simulink model "ChiefMaster_TTC580"  (R2022b)
settings: Solver=FixedStepAuto  StartTime=0.0  StopTime=10  FixedStep=0.01  RelTol=1e-3
values from neighbouring files (symbols this model uses):
  BattBox1_No = single(1)    [Parameters.m]
  BattBox2_No = single(2)    [Parameters.m]
  BattBox3_No = single(3)    [Parameters.m]
  CurrentLB = single(-3)    [Parameters.m]
  CurrentReductionConstant_Lvl0 = single(0.03)    [Parameters.m]
  CurrentReductionConstant_Lvl1 = single(0.05)    [Parameters.m]
  CurrentReductionConstant_Lvl2 = single(0.07)    [Parameters.m]
  CurrentReductionConstant_Lvl3 = single(0.1)    [Parameters.m]
  CurrentUB = single(3)    [Parameters.m]
  DCHV_Minus_In_Delay_ms = single(500)    [Parameters.m]
  FL_sHVC_CellBalanceVoltage_mV = single(3500)    [Parameters.m]
  FL_sInrushCurrent_dividebyzero = single(0.00001)    [Parameters.m]
  FL_u8HMI_BuzzerTimer = uint8(3)    [Parameters.m]
  IP_boActValue = true    [Parameters.m]
  IP_boDeactValue = false    [Parameters.m]
  IP_boInitValue = false    [Parameters.m]
  IP_s_LB = 18000    [Parameters.m]
  IP_s_UB = 22000    [Parameters.m]
  IP_sBatt1_ChargeCurrentMax_Factor = single(0.1)    [Parameters.m]
  IP_sBatt1_ChargeCurrentMax_LB = single(0)    [Parameters.m]
  IP_sBatt1_ChargeCurrentMax_Offset = single(0)    [Parameters.m]
  IP_sBatt1_ChargeCurrentMax_UB = single(6553.5)    [Parameters.m]
  IP_sBatt1_Current_Factor = single(0.1)    [Parameters.m]
  IP_sBatt1_Current_LB = single(-3276.8)    [Parameters.m]
  IP_sBatt1_Current_Offset = single(0)    [Parameters.m]
  IP_sBatt1_Current_UB = single(3276.8)    [Parameters.m]
  IP_sBatt1_DisChargeCurrentMax_Factor = single(0.1)    [Parameters.m]
  IP_sBatt1_DisChargeCurrentMax_LB = single(0)    [Parameters.m]
  IP_sBatt1_DisChargeCurrentMax_Offset = single(0)    [Parameters.m]
  IP_sBatt1_DisChargeCurrentMax_UB = single(6553.5)    [Parameters.m]
  IP_sBatt1_InsulationResistance_Factor = single(5)    [Parameters.m]
  IP_sBatt1_InsulationResistance_LB = single(0)    [Parameters.m]
  IP_sBatt1_InsulationResistance_Offset = single(0)    [Parameters.m]
  IP_sBatt1_InsulationResistance_UB = single(0)    [Parameters.m]
  IP_sBatt1_LiBa_IntResist_mOhm = single(25)    [Parameters.m]
  IP_sBatt1_SOC_Factor = single(1)    [Parameters.m]
  IP_sBatt1_SOC_LB = single(0)    [Parameters.m]
  IP_sBatt1_SOC_Offset = single(0)    [Parameters.m]
  IP_sBatt1_SOC_UB = single(100)    [Parameters.m]
  IP_sBatt1_SOH_Factor = single(1)    [Parameters.m]
  IP_sBatt1_SOH_LB = single(0)    [Parameters.m]
  IP_sBatt1_SOH_Offset = single(0)    [Parameters.m]
  IP_sBatt1_SOH_UB = single(100)    [Parameters.m]
  IP_sBatt1_Ubatt_Factor = single(0.1)    [Parameters.m]
  IP_sBatt1_Ubatt_LB = single(0)    [Parameters.m]
  IP_sBatt1_Ubatt_Offset = single(0)    [Parameters.m]
  IP_sBatt1_Ubatt_UB = single(6553.5)    [Parameters.m]
  IP_sBatt1_UserRi_Factor = single(1)    [Parameters.m]
  IP_sBatt1_UserRi_LB = single(0)    [Parameters.m]
  IP_sBatt1_UserRi_Offset = single(0)    [Parameters.m]
  IP_sBatt1_UserRi_UB = single(255)    [Parameters.m]
  IP_sBatt1_VoltageAtSensor_Factor = single(0.02)    [Parameters.m]
  IP_sBatt1_VoltageAtSensor_LB = single(0)    [Parameters.m]
  IP_sBatt1_VoltageAtSensor_Offset = single(0)    [Parameters.m]
  IP_sBatt1_VoltageAtSensor_UB = single(1310.7)    [Parameters.m]
  IP_sBatt2_LiBa_IntResist_mOhm = single(25)    [Parameters.m]
  IP_sBatt3_LiBa_IntResist_mOhm = single(25)    [Parameters.m]
  IP_sEM_LB = 2000    [Parameters.m]
  IP_sEM_UB = 8000    [Parameters.m]
  IP_sFB_LB = 5000    [Parameters.m]
  IP_sFB_UB = 10000    [Parameters.m]
  IP_sHVIL_LB = 12000    [Parameters.m]
  IP_sHVIL_UB = 15000    [Parameters.m]
  IP_sLoad_Voltage_Factor = single(1)    [Parameters.m]
  IP_sLoad_Voltage_LB = single(0)    [Parameters.m]
  IP_sLoad_Voltage_Offset = single(0)    [Parameters.m]
  IP_sLoad_Voltage_UB = single(65535)    [Parameters.m]
  IP_u8HVIL_Delay_ms = uint8(100)    [Parameters.m]
  IP_u8HW_IN_delay_ms = uint8(100)    [Parameters.m]
  IT_sInsulationSafeValue_kOhm = single(650)    [Parameters.m]
  IT_u8IMD_DelayTime_s = uint8(20)    [Parameters.m]
  MainHV_Minus_In_Delay = single(5)    [Parameters.m]
  MainHV_StatusDelay = single(5)    [Parameters.m]
  NotAvailable_uint16 = single(65535)    [Parameters.m]
  NotAvailable_uint8 = uint8(255)    [Parameters.m]
  OP_boHVIL_Supply = boolean(1)    [Parameters.m]
  SafeCurrentToCloseHV_A = single(5)    [Parameters.m]
  SafeVoltageToCloseHV_V = single(0.5)    [Parameters.m]
  UnexpectedBattChargingFcn_Available = boolean(1)    [Parameters.m]
  Voltage_NA_UB = uint16(65535)    [Parameters.m]
  VoltageSensorAvailableBB1 = boolean(0)    [Parameters.m]
  VoltageSensorAvailableBB2 = boolean(0)    [Parameters.m]
  VoltageSensorAvailableBB3 = boolean(0)    [Parameters.m]
libraries: simulink x184, Library_DataProcessing_v1_1 x167, Library_DataProcessing_v1 x142, libCM x28
(part 10 of 19)

== system ChiefMaster_TTC580/ChiefMaster/Flow Logic/System Status/SDError/Subsystem ==
  KL15_Reset : Inport
  BattPack_REL_Databus : Inport  Port=2
  BatteryPackSignals : Inport  Port=3
  AND : Logic  Inputs=3  AllPortsSameDT=off  OutDataTypeStr=boolean
  AND1 : Logic  Inputs=3  AllPortsSameDT=off  OutDataTypeStr=boolean
  AND2 : Logic  Inputs=3  AllPortsSameDT=off  OutDataTypeStr=boolean
  Bus Selector : BusSelector  OutputSignals=IT_BatterySignal_Databus.IT_sBMS_Current_BB1,IT_BatterySignal_Databus.IT_sBMS_Current_BB2,IT_BatterySignal_Databus.IT_sBMS_Current_BB3,IT_BatterySignal_Databus.IT_boBMS_SDError_BB1,IT_BatterySignal_Databus.IT_boBMS_SDError_BB2,IT_BatterySignal_Databus.IT_boBMS_SDError_BB3
  Bus Selector1 : BusSelector  OutputSignals=FL_boREQ_HV_ON_BB1,FL_boREQ_HV_ON_BB2,FL_boREQ_HV_ON_BB3
  Chart : Stateflow chart  TreatAsAtomicUnit=on
  Chart1 : Stateflow chart  TreatAsAtomicUnit=on
  Chart2 : Stateflow chart  TreatAsAtomicUnit=on
  Compare To Constant1 : simulink/Logic and Bit Operations/Compare To Constant  relop=>  const=1  OutDataTypeStr=boolean
  Compare To Constant2 : simulink/Logic and Bit Operations/Compare To Constant  relop===  const=0  OutDataTypeStr=boolean
  Compare To Constant3 : simulink/Logic and Bit Operations/Compare To Constant  relop=>  const=1  OutDataTypeStr=boolean
  Compare To Constant4 : simulink/Logic and Bit Operations/Compare To Constant  relop===  const=0  OutDataTypeStr=boolean
  Compare To Constant5 : simulink/Logic and Bit Operations/Compare To Constant  relop=>  const=1  OutDataTypeStr=boolean
  Compare To Constant6 : simulink/Logic and Bit Operations/Compare To Constant  relop===  const=0  OutDataTypeStr=boolean
  Detect Decrease : simulink/Logic and Bit Operations/Detect Decrease  vinit=0.0  OutDataTypeStr=boolean
  Detect Decrease1 : simulink/Logic and Bit Operations/Detect Decrease  vinit=0.0  OutDataTypeStr=boolean
  Detect Decrease2 : simulink/Logic and Bit Operations/Detect Decrease  vinit=0.0  OutDataTypeStr=boolean
  OR : Logic  Operator=OR  Inputs=3  AllPortsSameDT=off  OutDataTypeStr=boolean
  REL_Error_BB : Outport
  wires:
  BattPack_REL_Databus/1 -> Bus Selector1/1
  Bus Selector/1 -> Compare To Constant1/1  "<IT_sBMS_Current_BB1>"
  BatteryPackSignals/1 -> Bus Selector/1
  Compare To Constant6/1 -> Chart2/2(REQ_HV_ON_BB)
  Compare To Constant4/1 -> Chart1/2(REQ_HV_ON_BB)
  Compare To Constant2/1 -> Chart/2(REQ_HV_ON_BB)
  OR/1 -> REL_Error_BB/1
  AND2/1 -> OR/3
  AND1/1 -> OR/2
  KL15_Reset/1 -> Chart/3(KL15_CM_Reset), Chart1/3(KL15_CM_Reset), Chart2/3(KL15_CM_Reset)
  Chart2/1(Out) -> AND2/3
  Detect Decrease2/1 -> Chart2/1(In)
  Compare To Constant5/1 -> AND2/1
  Bus Selector/3 -> Compare To Constant5/1  "<IT_sBMS_Current_BB3>"
  Bus Selector/6 -> AND2/2  "<IT_boBMS_SDError_BB3>"
  Bus Selector1/3 -> Detect Decrease2/1, Compare To Constant6/1  "<FL_boREQ_HV_ON_BB3>"
  Bus Selector1/2 -> Compare To Constant4/1, Detect Decrease1/1  "<FL_boREQ_HV_ON_BB2>"
  Bus Selector/5 -> AND1/2  "<IT_boBMS_SDError_BB2>"
  Bus Selector/2 -> Compare To Constant3/1  "<IT_sBMS_Current_BB2>"
  Compare To Constant3/1 -> AND1/1
  Detect Decrease1/1 -> Chart1/1(In)
  Chart1/1(Out) -> AND1/3
  AND/1 -> OR/1
  Chart/1(Out) -> AND/3
  Detect Decrease/1 -> Chart/1(In)
  Compare To Constant1/1 -> AND/1
  Bus Selector/4 -> AND/2  "<IT_boBMS_SDError_BB1>"
  Bus Selector1/1 -> Compare To Constant2/1, Detect Decrease/1  "<FL_boREQ_HV_ON_BB1>"

== system ChiefMaster_TTC580/ChiefMaster/Flow Logic/System Status/SDError/Subsystem6 ==
  BatteryPackSignals : Inport
  AND3 : Logic  Operator=OR  Inputs=3  AllPortsSameDT=off  OutDataTypeStr=boolean
  Bus Selector2 : BusSelector  OutputSignals=IT_HW_Input_Databus.IT_boHW_Proximity_BB1,IT_HW_Input_Databus.IT_boHW_Proximity_BB2,IT_HW_Input_Databus.IT_boHW_Proximity_BB3
  Compare To Constant : simulink/Logic and Bit Operations/Compare To Constant  relop===  const=0  OutDataTypeStr=boolean
  Compare To Constant1 : simulink/Logic and Bit Operations/Compare To Constant  relop===  const=0  OutDataTypeStr=boolean
  Compare To Constant2 : simulink/Logic and Bit Operations/Compare To Constant  relop===  const=0  OutDataTypeStr=boolean
  SecuritySwitchError : Outport
  wires:
  Bus Selector2/2 -> Compare To Constant1/1  "<IT_boHW_Proximity_BB2>"
  AND3/1 -> SecuritySwitchError/1
  Bus Selector2/3 -> Compare To Constant2/1  "<IT_boHW_Proximity_BB3>"
  BatteryPackSignals/1 -> Bus Selector2/1
  Bus Selector2/1 -> Compare To Constant/1  "<IT_boHW_Proximity_BB1>"
  Compare To Constant/1 -> AND3/1
  Compare To Constant1/1 -> AND3/2
  Compare To Constant2/1 -> AND3/3

== system ChiefMaster_TTC580/ChiefMaster/Input Processing/Actia/Batt Box 1/Subsystem1 ==
  C_Batt1_ADS_3_560 : Inport
  C_Batt1_ADS_3_560_Timeout : Inport  Port=2
  Demux : Demux  Outputs=8
  Subsystem3 : Subsystem
  Terminator{,1..5} (6 alike) : Terminator
  IP_sActia_Batt1_Ubatt_Databus : Outport
  wires:
  C_Batt1_ADS_3_560/1 -> Demux/1
  Demux/2 -> Subsystem3/1(byte1)
  Demux/3 -> Subsystem3/2(byte2)
  Subsystem3/1(IP_sBatt1_Ubatt_Databus) -> IP_sActia_Batt1_Ubatt_Databus/1  "IP_sActia_Batt1_Ubatt_Databus"
  Demux/8 -> Terminator/1
  C_Batt1_ADS_3_560_Timeout/1 -> Subsystem3/3(C_Batt1_ADS_3_560_Timeout)
  Demux/7 -> Terminator1/1
  Demux/6 -> Terminator2/1
  Demux/5 -> Terminator3/1
  Demux/4 -> Terminator4/1
  Demux/1 -> Terminator5/1

== system ChiefMaster_TTC580/ChiefMaster/Input Processing/Actia/Batt Box 1/Subsystem13 ==
  C_Batt1_MyStatus_140_Timeout : Inport
  C_Batt1_Error_100_Timeout : Inport  Port=2
  C_Batt1_ADS_8_600_Timeout : Inport  Port=3
  C_Batt1_ADS_0_500_Timeout : Inport  Port=4
  C_Batt1_ADS_1_520_Timeout : Inport  Port=5
  C_Batt1_ADS_3_560_Timeout : Inport  Port=6
  AND : Logic  Inputs=6  AllPortsSameDT=off  OutDataTypeStr=boolean
  Constant : Constant
  Constant1 : Constant  Value=0
  NOT{,1..5} (6 alike) : Logic  Operator=NOT  AllPortsSameDT=off  OutDataTypeStr=boolean
  Switch : Switch  Criteria=u2 > Threshold  SaturateOnIntegerOverflow=off  InputSameDT=off
  IP_sActia_Batt1_Availability : Outport
  wires:
  Constant1/1 -> Switch/3
  Constant/1 -> Switch/1
  AND/1 -> Switch/2
  NOT4/1 -> AND/6
  NOT3/1 -> AND/5
  NOT2/1 -> AND/3
  NOT1/1 -> AND/2
  NOT/1 -> AND/1
  C_Batt1_ADS_1_520_Timeout/1 -> NOT3/1
  C_Batt1_ADS_8_600_Timeout/1 -> NOT2/1
  C_Batt1_Error_100_Timeout/1 -> NOT1/1
  C_Batt1_MyStatus_140_Timeout/1 -> NOT/1
  Switch/1 -> IP_sActia_Batt1_Availability/1  "IP_sActia_Batt1_Availability"
  C_Batt1_ADS_3_560_Timeout/1 -> NOT4/1
  C_Batt1_ADS_0_500_Timeout/1 -> NOT5/1
  NOT5/1 -> AND/4

== system ChiefMaster_TTC580/ChiefMaster/Input Processing/Actia/Batt Box 1/Subsystem2 ==
  C_Actia_Batt1_MyStatus_Msg : Inport
  C_Actia_Batt1_MyStatus_Timeout : Inport  Port=2
  Demux : Demux  Outputs=8
  NOT : Logic  Priority=5520  Operator=NOT  AllPortsSameDT=off  OutDataTypeStr=boolean
  Subsystem : Subsystem
  Subsystem2 : Subsystem
  Subsystem3 : Subsystem
  Subsystem4 : Subsystem
  Terminator : Terminator
  Batt1_MyStatus1_Databus : Outport
  IP_sActia_Batt1_ChargeCurrentMax_A_Databus : Outport  Port=2
  IP_sActia_Batt1_DisChargeCurrentMax_A_Databus : Outport  Port=3
  IP_sActia_Batt1_VoltageAtSensor_V_Databus : Outport  Port=4
  wires:
  C_Actia_Batt1_MyStatus_Msg/1 -> Demux/1
  Demux/1 -> Subsystem/1(byte1)
  Subsystem/1(Batt1_MyStatus1_Databus) -> Batt1_MyStatus1_Databus/1  "IP_Actia_Batt1_MyStatus1_Databus"
  Demux/2 -> Subsystem4/1(byte2)
  Demux/3 -> Subsystem4/2(byte3)
  Demux/4 -> Subsystem2/1(byte2)
  Demux/5 -> Subsystem2/2(byte3)
  Demux/6 -> Subsystem3/1(byte2)
  Demux/7 -> Subsystem3/2(byte3)
  Subsystem4/1(IP_sBatt1_ChargeCurrentMax_A_Databus) -> IP_sActia_Batt1_ChargeCurrentMax_A_Databus/1  "IP_sActia_Batt1_ChargeCurrentMax_A_Databus"
  Subsystem2/1(IP_sBatt1_DisChargeCurrentMax_A_Databus) -> IP_sActia_Batt1_DisChargeCurrentMax_A_Databus/1  "IP_sActia_Batt1_DisChargeCurrentMax_A_Databus"
  Subsystem3/1(IP_sBatt1_VoltageAtSensor_V_Databus) -> IP_sActia_Batt1_VoltageAtSensor_V_Databus/1  "IP_sActia_Batt1_VoltageAtSensor_V_Databus"
  Demux/8 -> Terminator/1
  C_Actia_Batt1_MyStatus_Timeout/1 -> NOT/1, Subsystem3/3(C_Actia_Batt1_MyStatus_Timeout), Subsystem2/3(C_Actia_Batt1_MyStatus_Timeout), Subsystem4/3(C_Actia_Batt1_MyStatus_Timeout)
  NOT/1 -> Subsystem/Enable

== system ChiefMaster_TTC580/ChiefMaster/Input Processing/Actia/Batt Box 1/Subsystem3 ==
  C_Batt1_ADS_0_500 : Inport
  C_Batt1_ADS_0_500_Timeout : Inport  Port=2
  Demux : Demux  Outputs=8
  Subsystem1 : Subsystem
  Subsystem2 : Subsystem
  Terminator{1..4} (4 alike) : Terminator
  IP_sActia_Batt1_MinCellVolt_mV_DataBus : Outport
  IP_sActia_Batt1_MaxCellVolt_mV_DataBus : Outport  Port=2
  wires:
  Subsystem2/1(IP_sActia_Batt1_MaxCellVolt_mV_DataBus) -> IP_sActia_Batt1_MaxCellVolt_mV_DataBus/1
  Subsystem1/1(IP_sActia_Batt1_MinCellVolt_mV_DataBus) -> IP_sActia_Batt1_MinCellVolt_mV_DataBus/1
  Demux/7 -> Subsystem2/2(byte7)
  Demux/6 -> Subsystem2/1(byte6)
  Demux/5 -> Subsystem1/2(byte5)
  Demux/4 -> Subsystem1/1(byte4)
  C_Batt1_ADS_0_500/1 -> Demux/1
  Demux/1 -> Terminator1/1
  Demux/2 -> Terminator2/1
  Demux/3 -> Terminator3/1
  C_Batt1_ADS_0_500_Timeout/1 -> Subsystem1/3(C_BMS500_Timeout), Subsystem2/3(C_BMS500_Timeout)
  Demux/8 -> Terminator4/1

== system ChiefMaster_TTC580/ChiefMaster/Input Processing/Actia/Batt Box 1/Subsystem4 ==
  C_Actia_Batt1_Error : Inport
  C_Actia_Batt1_Error_Timeout : Inport  Port=2
  Bus Creator : BusCreator  Inputs=7
  Bus Creator1 : BusCreator  Inputs=1
  Demux : Demux  Outputs=8
  NOT : Logic  Priority=5520  Operator=NOT  AllPortsSameDT=off  OutDataTypeStr=boolean
  Subsystem : Subsystem
  Subsystem1 : Subsystem
  Subsystem2 : Subsystem
  Terminator{1,3..6} (5 alike) : Terminator
  IP_Actia_sBatt1_MyStatus2_Databus : Outport
  IP_Actia_Batt1_Error_Databus : Outport  Port=2
  wires:
  Demux/8 -> Subsystem1/1(byte8)
  Bus Creator/1 -> IP_Actia_sBatt1_MyStatus2_Databus/1  "Batt1_MyStatus2_Databus"
  Demux/7 -> Subsystem/1(byte7)
  C_Actia_Batt1_Error/1 -> Demux/1
  Demux/1 -> Terminator1/1
  Demux/2 -> Subsystem2/1(byte2)
  Demux/3 -> Terminator3/1
  Demux/4 -> Terminator4/1
  Demux/5 -> Terminator5/1
  Demux/6 -> Terminator6/1
  C_Actia_Batt1_Error_Timeout/1 -> NOT/1
  NOT/1 -> Subsystem/Enable, Subsystem1/Enable, Subsystem2/Enable
  Subsystem/1(IP_boBatt1_HV_relay_PLUS_Sense) -> Bus Creator/1
  Subsystem/2(IP_boBatt1_HV_PRECHARGE_active) -> Bus Creator/2
  Subsystem/3(IP_boBatt1_HV_relay_MINUS_Sense) -> Bus Creator/3
  Subsystem/4(IP_boBatt1_IMD_active) -> Bus Creator/4
  Subsystem1/1(IP_boBatt1_Drive_Mode_active) -> Bus Creator/5
  Subsystem1/2(IP_boBatt1_PlugIn_Mode_active) -> Bus Creator/6
  Subsystem1/3(IP_boBatt1_Charging_finished) -> Bus Creator/7
  Subsystem2/1(IP_boBatt1_SDErr_SecuritySwitch) -> Bus Creator1/1
  Bus Creator1/1 -> IP_Actia_Batt1_Error_Databus/1  "Batt1_Error_Databus"

== system ChiefMaster_TTC580/ChiefMaster/Input Processing/Actia/Batt Box 1/Subsystem5 ==
  C_Batt1_ADS_8_600 : Inport
  C_Batt1_ADS_8_600_Timeout : Inport  Port=2
  Demux : Demux  Outputs=8
  Subsystem : Subsystem
  Subsystem1 : Subsystem
  Subsystem2 : Subsystem
  Subsystem3 : Subsystem
  Terminator1 : Terminator
  Terminator2 : Terminator
  Terminator3 : Terminator
  IP_sActia_Batt1_Current_A_DataBus : Outport
  IP_sActia_Batt1_InsulationResistance_kOhms_DataBus : Outport  Port=2
  IP_sActia_Batt1_SOC_percent_DataBus : Outport  Port=3
  IP_sActia_Batt1_SOH_percent_DataBus : Outport  Port=4
  wires:
  Demux/8 -> Subsystem3/1(byte8)
  Subsystem/1(IP_sBatt1_InsulationResistance_kOhms_DataBus) -> IP_sActia_Batt1_InsulationResistance_kOhms_DataBus/1  "IP_sActia_Batt1_InsulationResistance_kOhms_DataBus"
  Subsystem2/1(IP_sBatt1_Current_A_DataBus) -> IP_sActia_Batt1_Current_A_DataBus/1  "IP_sActia_Batt1_Current_A_DataBus"
  Demux/6 -> Subsystem/1(byte6)
  Demux/5 -> Subsystem2/2(byte5)
  Demux/4 -> Subsystem2/1(byte4)
  C_Batt1_ADS_8_600/1 -> Demux/1
  Demux/1 -> Terminator1/1
  Demux/2 -> Terminator2/1
  Demux/3 -> Terminator3/1
  C_Batt1_ADS_8_600_Timeout/1 -> Subsystem3/2(C_Batt1_ADS_8_600_Timeout), Subsystem1/2(C_Batt1_ADS_8_600_Timeout), Subsystem/2(C_Batt1_ADS_8_600_Timeout), Subsystem2/3(C_Batt1_ADS_8_600_Timeout)
  Demux/7 -> Subsystem1/1(byte7)
  Subsystem1/1(IP_sBatt1_SOC_percent_DataBus) -> IP_sActia_Batt1_SOC_percent_DataBus/1  "IP_sActia_Batt1_SOC_percent_DataBus"
  Subsystem3/1(IP_sBatt1_SOH_percent_DataBus) -> IP_sActia_Batt1_SOH_percent_DataBus/1  "IP_sActia_Batt1_SOH_percent_DataBus"

== system ChiefMaster_TTC580/ChiefMaster/Input Processing/Actia/Batt Box 1/Subsystem6 ==
  C_Batt1_ADS_1_520 : Inport
  C_Batt1_ADS_1_520_Timeout : Inport  Port=2
  Demux : Demux  Outputs=8
  Subsystem1 : Subsystem
  Subsystem2 : Subsystem
  Subsystem3 : Subsystem
  Terminator1 : Terminator
  Terminator2 : Terminator
  Terminator3 : Terminator
  IP_sActia_Batt1_UserRi_mOhms_DataBus : Outport
  IP_sActia_Batt1_MinTemp_degC_DataBus : Outport  Port=2
  IP_sActia_Batt1_MaxTemp_degC_DataBus : Outport  Port=3
  wires:
  Subsystem3/1(IP_sBatt1_UserRi_mOhms_DataBus) -> IP_sActia_Batt1_UserRi_mOhms_DataBus/1  "IP_sActia_Batt1_UserRi_mOhms_DataBus"
  C_Batt1_ADS_1_520_Timeout/1 -> Subsystem3/2(C_Batt1_ADS_8_600_Timeout), Subsystem2/3(C_BMS214_Timeout), Subsystem1/3(C_BMS214_Timeout)
  Demux/3 -> Terminator3/1
  Demux/2 -> Terminator2/1
  Demux/1 -> Terminator1/1
  C_Batt1_ADS_1_520/1 -> Demux/1
  Demux/8 -> Subsystem3/1(byte8)
  Demux/4 -> Subsystem1/1(byte4)
  Demux/5 -> Subsystem1/2(byte5)
  Demux/6 -> Subsystem2/1(byte6)
  Demux/7 -> Subsystem2/2(byte7)
  Subsystem1/1(IP_sBMS_MinTemp_degC_DataBus) -> IP_sActia_Batt1_MinTemp_degC_DataBus/1
  Subsystem2/1(IP_sBMS_MaxTemp_degC_DataBus) -> IP_sActia_Batt1_MaxTemp_degC_DataBus/1

== system ChiefMaster_TTC580/ChiefMaster/Input Processing/Actia/Batt Box 2/Subsystem1 ==
  C_Batt2_ADS_3_560 : Inport
  C_Batt2_ADS_3_560_Timeout : Inport  Port=2
  Demux : Demux  Outputs=8
  Subsystem3 : Subsystem
  Terminator{,1..5} (6 alike) : Terminator
  IP_sActia_Batt2_Ubatt_Databus : Outport
  wires:
  Demux/1 -> Terminator5/1
  Demux/4 -> Terminator4/1
  Demux/5 -> Terminator3/1
  Demux/6 -> Terminator2/1
  Demux/7 -> Terminator1/1
  C_Batt2_ADS_3_560_Timeout/1 -> Subsystem3/3(C_Batt2_ADS_3_560_Timeout)
  Demux/8 -> Terminator/1
  Subsystem3/1(IP_sBatt2_Ubatt_Databus) -> IP_sActia_Batt2_Ubatt_Databus/1  "IP_sActia_Batt2_Ubatt_Databus"
  Demux/3 -> Subsystem3/2(byte2)
  Demux/2 -> Subsystem3/1(byte1)
  C_Batt2_ADS_3_560/1 -> Demux/1

== system ChiefMaster_TTC580/ChiefMaster/Input Processing/Actia/Batt Box 2/Subsystem13 ==
  C_Batt2_MyStatus_140_Timeout : Inport
  C_Batt2_Error_100_Timeout : Inport  Port=2
  C_Batt2_ADS_8_600_Timeout : Inport  Port=3
  C_Batt2_ADS_501_Timeout : Inport  Port=4
  C_Batt2_ADS_1_520_Timeout : Inport  Port=5
  C_Batt2_ADS_3_560_Timeout : Inport  Port=6
  AND : Logic  Inputs=6  AllPortsSameDT=off  OutDataTypeStr=boolean
  Constant : Constant
  Constant1 : Constant  Value=0
  NOT{,1..5} (6 alike) : Logic  Operator=NOT  AllPortsSameDT=off  OutDataTypeStr=boolean
  Switch : Switch  Criteria=u2 > Threshold  SaturateOnIntegerOverflow=off  InputSameDT=off
  IP_sActia_Batt2_Availability : Outport
  wires:
  C_Batt2_ADS_3_560_Timeout/1 -> NOT4/1
  Switch/1 -> IP_sActia_Batt2_Availability/1  "IP_sActia_Batt2_Availability"
  C_Batt2_MyStatus_140_Timeout/1 -> NOT/1
  C_Batt2_Error_100_Timeout/1 -> NOT1/1
  C_Batt2_ADS_8_600_Timeout/1 -> NOT2/1
  C_Batt2_ADS_1_520_Timeout/1 -> NOT3/1
  NOT/1 -> AND/1
  NOT1/1 -> AND/2
  NOT2/1 -> AND/3
  NOT3/1 -> AND/5
  NOT4/1 -> AND/6
  AND/1 -> Switch/2
  Constant/1 -> Switch/1
  Constant1/1 -> Switch/3
  C_Batt2_ADS_501_Timeout/1 -> NOT5/1
  NOT5/1 -> AND/4

== system ChiefMaster_TTC580/ChiefMaster/Input Processing/Actia/Batt Box 2/Subsystem2 ==
  C_Actia_Batt2_MyStatus_Msg : Inport
  C_Actia_Batt2_MyStatus_Timeout : Inport  Port=2
  Demux : Demux  Outputs=8
  NOT : Logic  Priority=5520  Operator=NOT  AllPortsSameDT=off  OutDataTypeStr=boolean
  Subsystem : Subsystem
  Subsystem2 : Subsystem
  Subsystem3 : Subsystem
  Subsystem4 : Subsystem
  Terminator : Terminator
  Batt2_MyStatus1_Databus : Outport
  IP_sActia_Batt2_ChargeCurrentMax_A_Databus : Outport  Port=2
  IP_sActia_Batt2_DisChargeCurrentMax_A_Databus : Outport  Port=3
  IP_sActia_Batt2_VoltageAtSensor_V_Databus : Outport  Port=4
  wires:
  NOT/1 -> Subsystem/Enable
  C_Actia_Batt2_MyStatus_Timeout/1 -> Subsystem4/3(C_Actia_Batt2_MyStatus_Timeout), Subsystem2/3(C_Actia_Batt2_MyStatus_Timeout), Subsystem3/3(C_Actia_Batt2_MyStatus_Timeout), NOT/1
  Demux/8 -> Terminator/1
  Subsystem3/1(IP_sBatt2_VoltageAtSensor_V_Databus) -> IP_sActia_Batt2_VoltageAtSensor_V_Databus/1  "IP_sActia_Batt2_VoltageAtSensor_V_Databus"
  Subsystem2/1(IP_sBatt2_DisChargeCurrentMax_A_Databus) -> IP_sActia_Batt2_DisChargeCurrentMax_A_Databus/1  "IP_sActia_Batt2_DisChargeCurrentMax_A_Databus"
  Subsystem4/1(IP_sBatt2_ChargeCurrentMax_A_Databus) -> IP_sActia_Batt2_ChargeCurrentMax_A_Databus/1  "IP_sActia_Batt2_ChargeCurrentMax_A_Databus"
  Demux/7 -> Subsystem3/2(byte3)
  Demux/6 -> Subsystem3/1(byte2)
  Demux/5 -> Subsystem2/2(byte3)
  Demux/4 -> Subsystem2/1(byte2)
  Demux/3 -> Subsystem4/2(byte3)
  Demux/2 -> Subsystem4/1(byte2)
  Subsystem/1(Batt2_MyStatus1_Databus) -> Batt2_MyStatus1_Databus/1  "IP_Actia_Batt2_MyStatus1_Databus"
  Demux/1 -> Subsystem/1(byte1)
  C_Actia_Batt2_MyStatus_Msg/1 -> Demux/1

== system ChiefMaster_TTC580/ChiefMaster/Input Processing/Actia/Batt Box 2/Subsystem3 ==
  C_Batt1_ADS_0_500 : Inport
  C_Batt1_ADS_0_500_Timeout : Inport  Port=2
  Demux : Demux  Outputs=8
  Subsystem1 : Subsystem
  Subsystem2 : Subsystem
  Terminator{1..4} (4 alike) : Terminator
  IP_sActia_Batt2_MinCellVolt_mV_DataBus : Outport
  IP_sActia_Batt2_MaxCellVolt_mV_DataBus : Outport  Port=2
  wires:
  Subsystem2/1(IP_sActia_Batt2_MaxCellVolt_mV_DataBus) -> IP_sActia_Batt2_MaxCellVolt_mV_DataBus/1
  Subsystem1/1(IP_sActia_Batt2_MinCellVolt_mV_DataBus) -> IP_sActia_Batt2_MinCellVolt_mV_DataBus/1
  Demux/7 -> Subsystem2/2(byte7)
  Demux/6 -> Subsystem2/1(byte6)
  Demux/5 -> Subsystem1/2(byte5)
  Demux/4 -> Subsystem1/1(byte4)
  C_Batt1_ADS_0_500/1 -> Demux/1
  Demux/1 -> Terminator1/1
  Demux/2 -> Terminator2/1
  Demux/3 -> Terminator3/1
  C_Batt1_ADS_0_500_Timeout/1 -> Subsystem1/3(C_BMS500_Timeout), Subsystem2/3(C_BMS500_Timeout)
  Demux/8 -> Terminator4/1

== system ChiefMaster_TTC580/ChiefMaster/Input Processing/Actia/Batt Box 2/Subsystem4 ==
  C_Actia_Batt2_Error : Inport
  C_Actia_Batt2_Error_Timeout : Inport  Port=2
  Bus Creator : BusCreator  Inputs=7
  Bus Creator1 : BusCreator  Inputs=1
  Demux : Demux  Outputs=8
  NOT : Logic  Priority=5520  Operator=NOT  AllPortsSameDT=off  OutDataTypeStr=boolean
  Subsystem : Subsystem
  Subsystem1 : Subsystem
  Subsystem2 : Subsystem
  Terminator{1,3..6} (5 alike) : Terminator
  IP_Actia_sBatt2_MyStatus2_Databus : Outport
  IP_Actia_Batt2_Error_Databus : Outport  Port=2
  wires:
  Bus Creator1/1 -> IP_Actia_Batt2_Error_Databus/1  "Batt2_Error_Databus"
  Subsystem2/1(IP_boBatt2_SDErr_SecuritySwitch) -> Bus Creator1/1
  Subsystem1/3(IP_boBatt2_Charging_finished) -> Bus Creator/7
  Subsystem1/2(IP_boBatt2_PlugIn_Mode_active) -> Bus Creator/6
  Subsystem1/1(IP_boBatt2_Drive_Mode_active) -> Bus Creator/5
  Subsystem/4(IP_boBatt2_IMD_active) -> Bus Creator/4
  Subsystem/3(IP_boBatt2_HV_relay_MINUS_Sense) -> Bus Creator/3
  Subsystem/2(IP_boBatt2_HV_PRECHARGE_active) -> Bus Creator/2
  Subsystem/1(IP_boBatt2_HV_relay_PLUS_Sense) -> Bus Creator/1
  NOT/1 -> Subsystem2/Enable, Subsystem1/Enable, Subsystem/Enable
  C_Actia_Batt2_Error_Timeout/1 -> NOT/1
  Demux/6 -> Terminator6/1
  Demux/5 -> Terminator5/1
  Demux/4 -> Terminator4/1
  Demux/3 -> Terminator3/1
  Demux/2 -> Subsystem2/1(byte2)
  Demux/1 -> Terminator1/1
  C_Actia_Batt2_Error/1 -> Demux/1
  Demux/7 -> Subsystem/1(byte7)
  Bus Creator/1 -> IP_Actia_sBatt2_MyStatus2_Databus/1  "Batt2_MyStatus2_Databus"
  Demux/8 -> Subsystem1/1(byte8)

== system ChiefMaster_TTC580/ChiefMaster/Input Processing/Actia/Batt Box 2/Subsystem5 ==
  C_Batt2_ADS_8_600 : Inport
  C_Batt2_ADS_8_600_Timeout : Inport  Port=2
  Demux : Demux  Outputs=8
  Subsystem : Subsystem
  Subsystem1 : Subsystem
  Subsystem2 : Subsystem
  Subsystem3 : Subsystem
  Terminator1 : Terminator
  Terminator2 : Terminator
  Terminator3 : Terminator
  IP_sActia_Batt2_Current_A_DataBus : Outport
  IP_sActia_Batt2_InsulationResistance_kOhms_DataBus : Outport  Port=2
  IP_sActia_Batt2_SOC_percent_DataBus : Outport  Port=3
  IP_sActia_Batt2_SOH_percent_DataBus : Outport  Port=4
  wires:
  Subsystem3/1(IP_sBatt2_SOH_percent_DataBus) -> IP_sActia_Batt2_SOH_percent_DataBus/1  "IP_sActia_Batt2_SOH_percent_DataBus"
  Subsystem1/1(IP_sBatt2_SOC_percent_DataBus) -> IP_sActia_Batt2_SOC_percent_DataBus/1  "IP_sActia_Batt2_SOC_percent_DataBus"
  Demux/7 -> Subsystem1/1(byte7)
  C_Batt2_ADS_8_600_Timeout/1 -> Subsystem2/3(C_Batt2_ADS_8_600_Timeout), Subsystem/2(C_Batt2_ADS_8_600_Timeout), Subsystem1/2(C_Batt2_ADS_8_600_Timeout), Subsystem3/2(C_Batt2_ADS_8_600_Timeout)
  Demux/3 -> Terminator3/1
  Demux/2 -> Terminator2/1
  Demux/1 -> Terminator1/1
  C_Batt2_ADS_8_600/1 -> Demux/1
  Demux/4 -> Subsystem2/1(byte4)
  Demux/5 -> Subsystem2/2(byte5)
  Demux/6 -> Subsystem/1(byte6)
  Subsystem2/1(IP_sBatt2_Current_A_DataBus) -> IP_sActia_Batt2_Current_A_DataBus/1  "IP_sActia_Batt2_Current_A_DataBus"
  Subsystem/1(IP_sBatt2_InsulationResistance_kOhms_DataBus) -> IP_sActia_Batt2_InsulationResistance_kOhms_DataBus/1  "IP_sActia_Batt2_InsulationResistance_kOhms_DataBus"
  Demux/8 -> Subsystem3/1(byte8)

== system ChiefMaster_TTC580/ChiefMaster/Input Processing/Actia/Batt Box 2/Subsystem6 ==
  C_Batt2_ADS_1_520 : Inport
  C_Batt2_ADS_1_520_Timeout : Inport  Port=2
  Demux : Demux  Outputs=8
  Subsystem2 : Subsystem
  Subsystem3 : Subsystem
  Temp : Subsystem
  Terminator1 : Terminator
  Terminator2 : Terminator
  Terminator3 : Terminator
  IP_sActia_Batt2_UserRi_mOhms_DataBus : Outport
  IP_sActia_Batt2_MinTemp_degC_DataBus : Outport  Port=2
  IP_sActia_Batt2_MaxTemp_degC_DataBus : Outport  Port=3
  wires:
  Demux/7 -> Subsystem2/2(byte7)
  Demux/6 -> Subsystem2/1(byte6)
  Demux/5 -> Temp/2(byte5)
  Demux/4 -> Temp/1(byte4)
  Demux/8 -> Subsystem3/1(byte8)
  C_Batt2_ADS_1_520/1 -> Demux/1
  Demux/1 -> Terminator1/1
  Demux/2 -> Terminator2/1
  Demux/3 -> Terminator3/1
  C_Batt2_ADS_1_520_Timeout/1 -> Subsystem3/2(C_Batt2_ADS_8_600_Timeout), Subsystem2/3(C_BMS214_Timeout), Temp/3(C_BMS214_Timeout)
  Subsystem3/1(IP_sBatt2_UserRi_mOhms_DataBus) -> IP_sActia_Batt2_UserRi_mOhms_DataBus/1  "IP_sActia_Batt2_UserRi_mOhms_DataBus"
  Subsystem2/1(IP_sBMS_MaxTemp_degC_DataBus) -> IP_sActia_Batt2_MaxTemp_degC_DataBus/1
  Temp/1(IP_sBMS_MinTemp_degC_DataBus) -> IP_sActia_Batt2_MinTemp_degC_DataBus/1

== system ChiefMaster_TTC580/ChiefMaster/Input Processing/Actia/Batt Box 3/Subsystem1 ==
  C_Batt3_ADS_3_560 : Inport
  C_Batt3_ADS_3_560_Timeout : Inport  Port=2
  Demux : Demux  Outputs=8
  Subsystem3 : Subsystem
  Terminator{,1..5} (6 alike) : Terminator
  IP_sActia_Batt3_Ubatt_Databus : Outport
  wires:
  C_Batt3_ADS_3_560/1 -> Demux/1
  Demux/2 -> Subsystem3/1(byte1)
  Demux/3 -> Subsystem3/2(byte2)
  Subsystem3/1(IP_sBatt3_Ubatt_Databus) -> IP_sActia_Batt3_Ubatt_Databus/1  "IP_sActia_Batt3_Ubatt_Databus"
  Demux/8 -> Terminator/1
  C_Batt3_ADS_3_560_Timeout/1 -> Subsystem3/3(C_Batt3_ADS_3_560_Timeout)
  Demux/7 -> Terminator1/1
  Demux/6 -> Terminator2/1
  Demux/5 -> Terminator3/1
  Demux/4 -> Terminator4/1
  Demux/1 -> Terminator5/1

== system ChiefMaster_TTC580/ChiefMaster/Input Processing/Actia/Batt Box 3/Subsystem13 ==
  C_Batt3_MyStatus_140_Timeout : Inport
  C_Batt3_Error_100_Timeout : Inport  Port=2
  C_Batt3_ADS_8_600_Timeout : Inport  Port=3
  C_Batt2_ADS_0_Timeout : Inport  Port=4
  C_Batt3_ADS_1_520_Timeout : Inport  Port=5
  C_Batt3_ADS_3_560_Timeout : Inport  Port=6
  AND : Logic  Inputs=6  AllPortsSameDT=off  OutDataTypeStr=boolean
  Constant : Constant
  Constant1 : Constant  Value=0
  NOT{,1..5} (6 alike) : Logic  Operator=NOT  AllPortsSameDT=off  OutDataTypeStr=boolean
  Switch : Switch  Criteria=u2 > Threshold  SaturateOnIntegerOverflow=off  InputSameDT=off
  IP_sActia_Batt3_Availability : Outport
  wires:
  Constant1/1 -> Switch/3
  Constant/1 -> Switch/1
  AND/1 -> Switch/2
  NOT4/1 -> AND/6
  NOT3/1 -> AND/5
  NOT2/1 -> AND/3
  NOT1/1 -> AND/2
  NOT/1 -> AND/1
  C_Batt3_ADS_1_520_Timeout/1 -> NOT3/1
  C_Batt3_ADS_8_600_Timeout/1 -> NOT2/1
  C_Batt3_Error_100_Timeout/1 -> NOT1/1
  C_Batt3_MyStatus_140_Timeout/1 -> NOT/1
  Switch/1 -> IP_sActia_Batt3_Availability/1  "IP_sActia_Batt3_Availability"
  C_Batt3_ADS_3_560_Timeout/1 -> NOT4/1
  C_Batt2_ADS_0_Timeout/1 -> NOT5/1
  NOT5/1 -> AND/4

== system ChiefMaster_TTC580/ChiefMaster/Input Processing/Actia/Batt Box 3/Subsystem2 ==
  C_Actia_Batt3_MyStatus_Msg : Inport
  C_Actia_Batt3_MyStatus_Timeout : Inport  Port=2
  Demux : Demux  Outputs=8
  NOT : Logic  Priority=5520  Operator=NOT  AllPortsSameDT=off  OutDataTypeStr=boolean
  Subsystem : Subsystem
  Subsystem2 : Subsystem
  Subsystem3 : Subsystem
  Subsystem4 : Subsystem
  Terminator : Terminator
  Batt3_MyStatus1_Databus : Outport
  IP_sActia_Batt3_ChargeCurrentMax_A_Databus : Outport  Port=2
  IP_sActia_Batt3_DisChargeCurrentMax_A_Databus : Outport  Port=3
  IP_sActia_Batt3_VoltageAtSensor_V_Databus : Outport  Port=4
  wires:
  C_Actia_Batt3_MyStatus_Msg/1 -> Demux/1
  Demux/1 -> Subsystem/1(byte1)
  Subsystem/1(Batt3_MyStatus1_Databus) -> Batt3_MyStatus1_Databus/1  "IP_Actia_Batt3_MyStatus1_Databus"
  Demux/2 -> Subsystem4/1(byte2)
  Demux/3 -> Subsystem4/2(byte3)
  Demux/4 -> Subsystem2/1(byte2)
  Demux/5 -> Subsystem2/2(byte3)
  Demux/6 -> Subsystem3/1(byte2)
  Demux/7 -> Subsystem3/2(byte3)
  Subsystem4/1(IP_sBatt3_ChargeCurrentMax_A_Databus) -> IP_sActia_Batt3_ChargeCurrentMax_A_Databus/1  "IP_sActia_Batt3_ChargeCurrentMax_A_Databus"
  Subsystem2/1(IP_sBatt3_DisChargeCurrentMax_A_Databus) -> IP_sActia_Batt3_DisChargeCurrentMax_A_Databus/1  "IP_sActia_Batt3_DisChargeCurrentMax_A_Databus"
  Subsystem3/1(IP_sBatt3_VoltageAtSensor_V_Databus) -> IP_sActia_Batt3_VoltageAtSensor_V_Databus/1  "IP_sActia_Batt3_VoltageAtSensor_V_Databus"
  Demux/8 -> Terminator/1
  C_Actia_Batt3_MyStatus_Timeout/1 -> NOT/1, Subsystem3/3(C_Actia_Batt2_MyStatus_Timeout), Subsystem2/3(C_Actia_Batt2_MyStatus_Timeout), Subsystem4/3(C_Actia_Batt2_MyStatus_Timeout)
  NOT/1 -> Subsystem/Enable

== system ChiefMaster_TTC580/ChiefMaster/Input Processing/Actia/Batt Box 3/Subsystem3 ==
  C_Batt1_ADS_0_500 : Inport
  C_Batt1_ADS_0_500_Timeout : Inport  Port=2
  Demux : Demux  Outputs=8
  Subsystem1 : Subsystem
  Subsystem2 : Subsystem
  Terminator{1..4} (4 alike) : Terminator
  IP_sActia_Batt3_MinCellVolt_mV_DataBus : Outport
  IP_sActia_Batt3_MaxCellVolt_mV_DataBus : Outport  Port=2
  wires:
  Subsystem2/1(IP_sActia_Batt3_MaxCellVolt_mV_DataBus) -> IP_sActia_Batt3_MaxCellVolt_mV_DataBus/1
  Subsystem1/1(IP_sActia_Batt3_MinCellVolt_mV_DataBus) -> IP_sActia_Batt3_MinCellVolt_mV_DataBus/1
  Demux/7 -> Subsystem2/2(byte7)
  Demux/6 -> Subsystem2/1(byte6)
  Demux/5 -> Subsystem1/2(byte5)
  Demux/4 -> Subsystem1/1(byte4)
  C_Batt1_ADS_0_500/1 -> Demux/1
  Demux/1 -> Terminator1/1
  Demux/2 -> Terminator2/1
  Demux/3 -> Terminator3/1
  C_Batt1_ADS_0_500_Timeout/1 -> Subsystem1/3(C_BMS500_Timeout), Subsystem2/3(C_BMS500_Timeout)
  Demux/8 -> Terminator4/1

== system ChiefMaster_TTC580/ChiefMaster/Input Processing/Actia/Batt Box 3/Subsystem4 ==
  C_Actia_Batt3_Error : Inport
  C_Actia_Batt3_Error_Timeout : Inport  Port=2
  Bus Creator : BusCreator  Inputs=7
  Bus Creator1 : BusCreator  Inputs=1
  Demux : Demux  Outputs=8
  NOT : Logic  Priority=5520  Operator=NOT  AllPortsSameDT=off  OutDataTypeStr=boolean
  Subsystem : Subsystem
  Subsystem1 : Subsystem
  Subsystem2 : Subsystem
  Terminator{1,3..6} (5 alike) : Terminator
  IP_Actia_sBatt3_MyStatus2_Databus : Outport
  IP_Actia_Batt3_Error_Databus : Outport  Port=2
  wires:
  Demux/8 -> Subsystem1/1(byte8)
  Bus Creator/1 -> IP_Actia_sBatt3_MyStatus2_Databus/1  "Batt3_MyStatus2_Databus"
  Demux/7 -> Subsystem/1(byte7)
  C_Actia_Batt3_Error/1 -> Demux/1
  Demux/1 -> Terminator1/1
  Demux/2 -> Subsystem2/1(byte2)
  Demux/3 -> Terminator3/1
  Demux/4 -> Terminator4/1
  Demux/5 -> Terminator5/1
  Demux/6 -> Terminator6/1
  C_Actia_Batt3_Error_Timeout/1 -> NOT/1
  NOT/1 -> Subsystem/Enable, Subsystem1/Enable, Subsystem2/Enable
  Subsystem/1(IP_boBatt3_HV_relay_PLUS_Sense) -> Bus Creator/1
  Subsystem/2(IP_boBatt3_HV_PRECHARGE_active) -> Bus Creator/2
  Subsystem/3(IP_boBatt3_HV_relay_MINUS_Sense) -> Bus Creator/3
  Subsystem/4(IP_boBatt3_IMD_active) -> Bus Creator/4
  Subsystem1/1(IP_boBatt3_Drive_Mode_active) -> Bus Creator/5
  Subsystem1/2(IP_boBatt3_PlugIn_Mode_active) -> Bus Creator/6
  Subsystem1/3(IP_boBatt3_Charging_finished) -> Bus Creator/7
  Subsystem2/1(IP_boBatt3_SDErr_SecuritySwitch) -> Bus Creator1/1
  Bus Creator1/1 -> IP_Actia_Batt3_Error_Databus/1  "Batt3_Error_Databus"

== system ChiefMaster_TTC580/ChiefMaster/Input Processing/Actia/Batt Box 3/Subsystem5 ==
  C_Batt3_ADS_8_600 : Inport
  C_Batt3_ADS_8_600_Timeout : Inport  Port=2
  Demux : Demux  Outputs=8
  Subsystem : Subsystem
  Subsystem1 : Subsystem
  Subsystem2 : Subsystem
  Subsystem3 : Subsystem
  Terminator1 : Terminator
  Terminator2 : Terminator
  Terminator3 : Terminator
  IP_sActia_Batt3_Current_A_DataBus : Outport
  IP_sActia_Batt3_InsulationResistance_kOhms_DataBus : Outport  Port=2
  IP_sActia_Batt3_SOC_percent_DataBus : Outport  Port=3
  IP_sActia_Batt3_SOH_percent_DataBus : Outport  Port=4
  wires:
  Demux/8 -> Subsystem3/1(byte8)
  Subsystem/1(IP_sBatt3_InsulationResistance_kOhms_DataBus) -> IP_sActia_Batt3_InsulationResistance_kOhms_DataBus/1  "IP_sActia_Batt3_InsulationResistance_kOhms_DataBus"
  Subsystem2/1(IP_sBatt3_Current_A_DataBus) -> IP_sActia_Batt3_Current_A_DataBus/1  "IP_sActia_Batt3_Current_A_DataBus"
  Demux/6 -> Subsystem/1(byte6)
  Demux/5 -> Subsystem2/2(byte5)
  Demux/4 -> Subsystem2/1(byte4)
  C_Batt3_ADS_8_600/1 -> Demux/1
  Demux/1 -> Terminator1/1
  Demux/2 -> Terminator2/1
  Demux/3 -> Terminator3/1
  C_Batt3_ADS_8_600_Timeout/1 -> Subsystem3/2(C_Batt3_ADS_8_600_Timeout), Subsystem1/2(C_Batt3_ADS_8_600_Timeout), Subsystem/2(C_Batt3_ADS_8_600_Timeout), Subsystem2/3(C_Batt3_ADS_8_600_Timeout)
  Demux/7 -> Subsystem1/1(byte7)
  Subsystem1/1(IP_sBatt3_SOC_percent_DataBus) -> IP_sActia_Batt3_SOC_percent_DataBus/1  "IP_sActia_Batt3_SOC_percent_DataBus"
  Subsystem3/1(IP_sBatt3_SOH_percent_DataBus) -> IP_sActia_Batt3_SOH_percent_DataBus/1  "IP_sActia_Batt3_SOH_percent_DataBus"

== system ChiefMaster_TTC580/ChiefMaster/Input Processing/Actia/Batt Box 3/Subsystem6 ==
  C_Batt3_ADS_1_520 : Inport
  C_Batt3_ADS_1_520_Timeout : Inport  Port=2
  Demux : Demux  Outputs=8
  Subsystem1 : Subsystem
  Subsystem2 : Subsystem
  Subsystem3 : Subsystem
  Terminator1 : Terminator
  Terminator2 : Terminator
  Terminator3 : Terminator
  IP_sActia_Batt3_UserRi_mOhms_DataBus : Outport
  IP_sActia_Batt3_MinTemp_degC_DataBus : Outport  Port=2
  IP_sActia_Batt3_MaxTemp_degC_DataBus : Outport  Port=3
  wires:
  Subsystem3/1(IP_sBatt3_UserRi_mOhms_DataBus) -> IP_sActia_Batt3_UserRi_mOhms_DataBus/1  "IP_sActia_Batt3_UserRi_mOhms_DataBus"
  C_Batt3_ADS_1_520_Timeout/1 -> Subsystem3/2(C_Batt3_ADS_8_600_Timeout), Subsystem2/3(C_BMS214_Timeout), Subsystem1/3(C_BMS214_Timeout)
  Demux/3 -> Terminator3/1
  Demux/2 -> Terminator2/1
  Demux/1 -> Terminator1/1
  C_Batt3_ADS_1_520/1 -> Demux/1
  Demux/8 -> Subsystem3/1(byte8)
  Demux/4 -> Subsystem1/1(byte4)
  Demux/5 -> Subsystem1/2(byte5)
  Demux/6 -> Subsystem2/1(byte6)
  Demux/7 -> Subsystem2/2(byte7)
  Subsystem1/1(IP_sBMS_MinTemp_degC_DataBus) -> IP_sActia_Batt3_MinTemp_degC_DataBus/1
  Subsystem2/1(IP_sBMS_MaxTemp_degC_DataBus) -> IP_sActia_Batt3_MaxTemp_degC_DataBus/1

== system ChiefMaster_TTC580/ChiefMaster/Input Processing/LiBa/LiBa_Box1/BMS_CellTemperature ==
  C_LB_Batt1_CellTemperature_Msg : Inport
  C_LB_Batt1_CellTemperature_Timeout : Inport  Port=2
  Bus Creator1 : BusCreator  Inputs=7
  Demux : Demux  Outputs=8
  Subsystem : Subsystem
  Subsystem1 : Subsystem
  Subsystem2 : Subsystem
  Subsystem3 : Subsystem
  Subsystem4 : Subsystem
  Subsystem5 : Subsystem
  Subsystem6 : Subsystem
  Terminator1 : Terminator
  IP_LB_Batt1_CellTemperature_DataBus : Outport
  wires:
  Subsystem3/1(IP_LB_BMS_ACT_Cel_T_Min_Cel_DataBus) -> Bus Creator1/4
  [C_LB_BMS_CellTemperature_Timeout] -> Subsystem3/2(C_LB_BMS_CellTemperature_Timeout)
  Demux/4 -> Subsystem3/1(byte3)
  Demux/3 -> Subsystem2/1(byte2)
  Demux/2 -> Subsystem1/1(byte1)
  C_LB_Batt1_CellTemperature_Msg/1 -> Demux/1
  Demux/1 -> Subsystem/1(byte0)
  C_LB_Batt1_CellTemperature_Timeout/1 -> [C_LB_BMS_CellTemperature_Timeout]
  [C_LB_BMS_CellTemperature_Timeout] -> Subsystem/2(C_LB_BMS_CellTemperature_Timeout)
  [C_LB_BMS_CellTemperature_Timeout] -> Subsystem1/2(C_LB_BMS_CellTemperature_Timeout)
  [C_LB_BMS_CellTemperature_Timeout] -> Subsystem2/2(C_LB_BMS_CellTemperature_Timeout)
  Demux/8 -> Terminator1/1
  Subsystem/1(IP_LB_BMS_ACT_Cel_T_Avg_DataBus) -> Bus Creator1/1
  Subsystem1/1(IP_LB_BMS_ACT_Cel_T_Min_Value_DataBus) -> Bus Creator1/2
  Subsystem2/1(IP_LB_BMS_ACT_Cel_T_Max_Value_DataBus) -> Bus Creator1/3
  Bus Creator1/1 -> IP_LB_Batt1_CellTemperature_DataBus/1  "IP_LB_Batt1_CellTemperature_DataBus"
  [C_LB_BMS_CellTemperature_Timeout] -> Subsystem4/2(C_LB_BMS_CellTemperature_Timeout)
  [C_LB_BMS_CellTemperature_Timeout] -> Subsystem5/2(C_LB_BMS_CellTemperature_Timeout)
  [C_LB_BMS_CellTemperature_Timeout] -> Subsystem6/2(C_LB_BMS_CellTemperature_Timeout)
  Demux/5 -> Subsystem4/1(byte1)
  Demux/6 -> Subsystem5/1(byte2)
  Demux/7 -> Subsystem6/1(byte3)
  Subsystem4/1(IP_LB_BMS_ACT_Cel_T_Min_CMU_DataBus) -> Bus Creator1/5
  Subsystem5/1(IP_LB_BMS_ACT_Cel_T_Max_Cel_DataBus) -> Bus Creator1/6
  Subsystem6/1(IP_LB_BMS_ACT_Cel_V_Max_Cel_DataBus) -> Bus Creator1/7

== system ChiefMaster_TTC580/ChiefMaster/Input Processing/LiBa/LiBa_Box1/BMS_CellVoltage01 ==
  C_LB_Batt1_CellVoltage01_Msg : Inport
  C_LB_Batt1_CellVoltage01_Timeout : Inport  Port=2
  Bus Creator1 : BusCreator  Inputs=3
  Demux : Demux  Outputs=8
  Subsystem : Subsystem
  Subsystem1 : Subsystem
  Subsystem2 : Subsystem
  Terminator : Terminator
  Terminator1 : Terminator
  IP_LB_Batt1_CellVoltage01_DataBus : Outport
  wires:
  C_LB_Batt1_CellVoltage01_Msg/1 -> Demux/1
  Demux/1 -> Subsystem/1(byte0)
  Demux/2 -> Subsystem/2(byte1)
  C_LB_Batt1_CellVoltage01_Timeout/1 -> [C_LB_BMS_CellVoltage01_Timeout]
  [C_LB_BMS_CellVoltage01_Timeout] -> Subsystem/3(C_LB_CellVoltage01_Timeout)
  Demux/3 -> Subsystem1/1(byte2)
  Demux/4 -> Subsystem1/2(byte3)
  [C_LB_BMS_CellVoltage01_Timeout] -> Subsystem1/3(C_LB_CellVoltage01_Timeout)
  Demux/5 -> Subsystem2/1(byte4)
  Demux/6 -> Subsystem2/2(byte5)
  [C_LB_BMS_CellVoltage01_Timeout] -> Subsystem2/3(C_LB_CellVoltage01_Timeout)
  Demux/7 -> Terminator/1
  Demux/8 -> Terminator1/1
  Subsystem/1(IP_LB_BMS_ACT_Cel_mV_Min_DataBus) -> Bus Creator1/1
  Subsystem1/1(IP_LB_BMS_ACT_Cel_mV_AVG_DataBus) -> Bus Creator1/2
  Subsystem2/1(IP_LB_BMS_ACT_Cel_mV_Max_DataBus) -> Bus Creator1/3
  Bus Creator1/1 -> IP_LB_Batt1_CellVoltage01_DataBus/1  "IP_LB_Batt1_CellVoltage01_DataBus"

== system ChiefMaster_TTC580/ChiefMaster/Input Processing/LiBa/LiBa_Box1/BMS_CellVoltageNumber ==
  C_LB_Batt1_CellVoltage02_Msg : Inport
  C_LB_Batt1_CellVoltage02_Timeout : Inport  Port=2
  Bus Creator1 : BusCreator  Inputs=4
  Demux : Demux  Outputs=8
  Subsystem : Subsystem
  Subsystem1 : Subsystem
  Subsystem2 : Subsystem
  Subsystem3 : Subsystem
  Terminator{,1..3} (4 alike) : Terminator
  IP_LB_Batt1_CellVoltage02_DataBus : Outport
  wires:
  Bus Creator1/1 -> IP_LB_Batt1_CellVoltage02_DataBus/1  "IP_LB_Batt1_CellVoltage02_DataBus"
  Subsystem2/1(IP_LB_BMS_ACT_Cel_V_Max_Cel_DataBus) -> Bus Creator1/3
  Subsystem1/1(IP_LB_BMS_ACT_Cel_V_Min_CMU_DataBus) -> Bus Creator1/2
  Subsystem/1(IP_LB_BMS_ACT_Cel_V_Min_Cel_DataBus) -> Bus Creator1/1
  Demux/8 -> Terminator1/1
  Demux/7 -> Terminator/1
  [C_LB_BMS_CellVoltage02_Timeout] -> Subsystem2/2(C_LB_CellVoltage02_Timeout)
  [C_LB_BMS_CellVoltage02_Timeout] -> Subsystem1/2(C_LB_CellVoltage02_Timeout)
  [C_LB_BMS_CellVoltage02_Timeout] -> Subsystem/2(C_LB_CellVoltage02_Timeout)
  C_LB_Batt1_CellVoltage02_Timeout/1 -> [C_LB_BMS_CellVoltage02_Timeout]
  Demux/1 -> Subsystem/1(byte0)
  C_LB_Batt1_CellVoltage02_Msg/1 -> Demux/1
  Demux/2 -> Subsystem1/1(byte1)
  Demux/3 -> Subsystem2/1(byte2)
  Demux/4 -> Subsystem3/1(byte3)
  [C_LB_BMS_CellVoltage02_Timeout] -> Subsystem3/2(C_LB_CellVoltage02_Timeout)
  Subsystem3/1(IP_LB_BMS_ACT_Cel_V_Max_CMU_DataBus) -> Bus Creator1/4
  Demux/6 -> Terminator2/1
  Demux/5 -> Terminator3/1

== system ChiefMaster_TTC580/ChiefMaster/Input Processing/LiBa/LiBa_Box1/BMS_InsulationMonitor ==
  C_LB_Batt1_InsulationMonitor_Msg : Inport
  C_LB_Batt1_InsulationMonitor_Timeout : Inport  Port=2
  Bus Creator1 : BusCreator  Inputs=3
  Demux : Demux  Outputs=8
  Subsystem : Subsystem
  Subsystem1 : Subsystem
  Subsystem2 : Subsystem
  Terminator : Terminator
  Terminator1 : Terminator
  IP_LB_Batt1_InsulationMonitor_DataBus : Outport
  wires:
  Bus Creator1/1 -> IP_LB_Batt1_InsulationMonitor_DataBus/1  "IP_LB_Batt1_InsulationMonitor_DataBus"
  Subsystem2/1(IP_LB_BMS_Pack_Leak_Mid_Raw_mV_DataBus) -> Bus Creator1/3
  Subsystem1/1(IP_LB_BMS_Pack_Leak_Neg_Raw_mV_DataBus) -> Bus Creator1/2
  Subsystem/1(IP_LB_BMS_Pack_Leak_Pos_Raw_mV_DataBus) -> Bus Creator1/1
  Demux/8 -> Terminator1/1
  Demux/7 -> Terminator/1
  [C_LB_BMS_InsulationMonitor_Timeout] -> Subsystem2/3(C_LB_BMS_InsulationMonitor_Timeout)
  Demux/6 -> Subsystem2/2(byte5)
  Demux/5 -> Subsystem2/1(byte4)
  [C_LB_BMS_InsulationMonitor_Timeout] -> Subsystem1/3(C_LB_BMS_InsulationMonitor_Timeout)
  Demux/4 -> Subsystem1/2(byte3)
  Demux/3 -> Subsystem1/1(byte2)
  [C_LB_BMS_InsulationMonitor_Timeout] -> Subsystem/3(C_LB_BMS_InsulationMonitor_Timeout)
  C_LB_Batt1_InsulationMonitor_Timeout/1 -> [C_LB_BMS_InsulationMonitor_Timeout]
  Demux/2 -> Subsystem/2(byte1)
  Demux/1 -> Subsystem/1(byte0)
  C_LB_Batt1_InsulationMonitor_Msg/1 -> Demux/1

== system ChiefMaster_TTC580/ChiefMaster/Input Processing/LiBa/LiBa_Box1/BMS_Status01 ==
  C_LB_Batt1_Status01_Msg : Inport
  C_LB_Batt1_Status01_Timeout : Inport  Port=2
  Bus Creator1 : BusCreator  Inputs=9
  Demux : Demux  Outputs=8
  Extract Bits : simulink/Logic and Bit Operations/Extract Bits  bitsToExtract=Range of bits  numBits=8  bitIdxRange=[0 3]  outScalingMode=Preserve fixed-point scaling
  Extract Bits1 : simulink/Logic and Bit Operations/Extract Bits  bitsToExtract=Range of bits  numBits=8  bitIdxRange=[4]  outScalingMode=Preserve fixed-point scaling
  Extract Bits2 : simulink/Logic and Bit Operations/Extract Bits  bitsToExtract=Range of bits  numBits=8  bitIdxRange=[5]  outScalingMode=Preserve fixed-point scaling
  Extract Bits3 : simulink/Logic and Bit Operations/Extract Bits  bitsToExtract=Range of bits  numBits=8  bitIdxRange=[6]  outScalingMode=Preserve fixed-point scaling
  Extract Bits4 : simulink/Logic and Bit Operations/Extract Bits  bitsToExtract=Range of bits  numBits=8  bitIdxRange=[7]  outScalingMode=Preserve fixed-point scaling
  Lib_InputProcessing_dflt0_flag{,1..3} (4 alike) : Library_DataProcessing_v1_1/Lib_InputProcessing_dflt0_flag  SystemSampleTime=-1  VariantActivationTime=update diagram  Latency=0  AutoFrameSizeCalculation=off
  Lib_InputProcessing_state : Library_DataProcessing_v1_1/Lib_InputProcessing_state  SystemSampleTime=-1  VariantActivationTime=update diagram  Latency=0  AutoFrameSizeCalculation=off
  NOT{1..5} (5 alike) : Logic  Operator=NOT  AllPortsSameDT=off  OutDataTypeStr=boolean
  Subsystem1 : Subsystem
  Subsystem2 : Subsystem
  Subsystem3 : Subsystem
  Subsystem4 : Subsystem
  Terminator2 : Terminator
  IP_LB_Batt1_Status01_DataBus : Outport
  wires:
  Bus Creator1/1 -> IP_LB_Batt1_Status01_DataBus/1  "IP_LB_Batt1_Status01_DataBus"
  Subsystem2/1(IP_LB_BMS_IO_State_Output_DataBus) -> Bus Creator1/7
  Subsystem1/1(IP_LB_BMS_IO_state_Input_DataBus) -> Bus Creator1/6
  Lib_InputProcessing_state/1 -> Bus Creator1/1  "IP_u8LB_BMS_Status"
  [C_LB_BMS_Status01_Timeout] -> Subsystem2/2(C_LB_BMS_Status01_Timeout)
  [C_LB_BMS_Status01_Timeout] -> Subsystem1/2(C_LB_BMS_Status01_Timeout)
  [C_LB_BMS_Status01_Timeout] -> NOT1/1
  C_LB_Batt1_Status01_Timeout/1 -> [C_LB_BMS_Status01_Timeout]
  Demux/1 -> Extract Bits4/1, Extract Bits3/1, Extract Bits2/1, Extract Bits1/1, Extract Bits/1
  C_LB_Batt1_Status01_Msg/1 -> Demux/1
  Demux/2 -> Subsystem1/1(byte1)
  Demux/3 -> Subsystem2/1(byte2)
  [C_LB_BMS_Status01_Timeout] -> Subsystem3/3(C_LB_BMS_Status01_Timeout)
  Subsystem3/1(IP_LB_BMS_DYN_Lim_Current_IN_A_DataBus) -> Bus Creator1/8
  Extract Bits/1 -> Lib_InputProcessing_state/1
  Extract Bits1/1 -> Lib_InputProcessing_dflt0_flag/1
  Lib_InputProcessing_dflt0_flag/1 -> Bus Creator1/2  "IP_boLB_BMS_FlagsChargerActive"
  [C_LB_BMS_Status01_Timeout] -> NOT2/1
  [C_LB_BMS_Status01_Timeout] -> NOT3/1
  Extract Bits2/1 -> Lib_InputProcessing_dflt0_flag1/1
  Extract Bits3/1 -> Lib_InputProcessing_dflt0_flag2/1
  [C_LB_BMS_Status01_Timeout] -> NOT4/1
  [C_LB_BMS_Status01_Timeout] -> NOT5/1
  Extract Bits4/1 -> Lib_InputProcessing_dflt0_flag3/1
  Lib_InputProcessing_dflt0_flag1/1 -> Bus Creator1/3  "IP_boLB_BMS_FlagsLoadActive"
  Lib_InputProcessing_dflt0_flag2/1 -> Bus Creator1/4  "IP_boLB_BMS_FlagsPreChargeActive"
  Lib_InputProcessing_dflt0_flag3/1 -> Bus Creator1/5  "IP_boLB_BMS_FlagsBalancingActive"
  Demux/4 -> Terminator2/1
  Demux/5 -> Subsystem3/1(byte4)
  Demux/6 -> Subsystem3/2(byte5)
  Subsystem4/1(IP_LB_BMS_DYN_Lim_Current_OUT_A_DataBus) -> Bus Creator1/9
  Demux/7 -> Subsystem4/1(byte6)
  Demux/8 -> Subsystem4/2(byte7)
  [C_LB_BMS_Status01_Timeout] -> Subsystem4/3(C_LB_BMS_Status01_Timeout)
  NOT1/1 -> Lib_InputProcessing_state/Enable
  NOT2/1 -> Lib_InputProcessing_dflt0_flag/Enable
  NOT3/1 -> Lib_InputProcessing_dflt0_flag1/Enable
  NOT4/1 -> Lib_InputProcessing_dflt0_flag2/Enable
  NOT5/1 -> Lib_InputProcessing_dflt0_flag3/Enable

== system ChiefMaster_TTC580/ChiefMaster/Input Processing/LiBa/LiBa_Box1/BMS_Status02 ==
  C_LB_Batt1_Status02_Msg : Inport
  C_LB_Batt1_Status02_Timeout : Inport  Port=2
  Bus Creator1 : BusCreator  Inputs=3
  Demux : Demux  Outputs=8
  Subsystem1 : Subsystem
  Subsystem2 : Subsystem
  Subsystem3 : Subsystem
  IP_LB_Batt1_Status02_DataBus : Outport
  wires:
  [C_LB_BMS_Status02_Timeout] -> Subsystem3/3(C_LB_BMS_Status02_Timeout)
  C_LB_Batt1_Status02_Msg/1 -> Demux/1
  C_LB_Batt1_Status02_Timeout/1 -> [C_LB_BMS_Status02_Timeout]
  Bus Creator1/1 -> IP_LB_Batt1_Status02_DataBus/1  "IP_LB_Batt1_Status02_DataBus"
  Demux/1 -> Subsystem3/1(byte0)
  Demux/2 -> Subsystem3/2(byte1)
  Subsystem3/1(IP_LB_BMS_Pack_Q_SOC_Internal_DataBus) -> Bus Creator1/1
  Demux/3 -> Subsystem1/1(byte2)
  Demux/5 -> Subsystem1/3(byte4)
  Demux/6 -> Subsystem1/4(byte5)
  [C_LB_BMS_Status02_Timeout] -> Subsystem1/5(C_LB_BMS_Status02_Timeout)
  Demux/4 -> Subsystem1/2(byte3)
  Subsystem1/1(IP_LB_BMS_Pack_Current_Master_mA_DataBus) -> Bus Creator1/2
  [C_LB_BMS_Status02_Timeout] -> Subsystem2/3(C_LB_BMS_Status02_Timeout)
  Demux/8 -> Subsystem2/2(byte7)
  Demux/7 -> Subsystem2/1(byte6)
  Subsystem2/1(IP_LB_BMS_Pack_V_Cells_DataBus) -> Bus Creator1/3

== system ChiefMaster_TTC580/ChiefMaster/Input Processing/LiBa/LiBa_Box1/BMS_Status03 ==
  C_LB_Batt1_Status03_Msg : Inport
  C_LB_Batt1_Status03_Timeout : Inport  Port=2
  Bus Creator1 : BusCreator  Inputs=1
  Demux : Demux  Outputs=8
  Subsystem3 : Subsystem
  Terminator{,1..5} (6 alike) : Terminator
  IP_LB_Batt1_Status03_DataBus : Outport
  wires:
  Subsystem3/1(IP_LB_BMS_REQ_Charger_Current_A_DataBus) -> Bus Creator1/1
  Demux/2 -> Subsystem3/2(byte1)
  Demux/1 -> Subsystem3/1(byte0)
  Bus Creator1/1 -> IP_LB_Batt1_Status03_DataBus/1  "IP_LB_Batt1_Status03_DataBus"
  C_LB_Batt1_Status03_Timeout/1 -> [C_LB_BMS_Status03_Timeout]
  C_LB_Batt1_Status03_Msg/1 -> Demux/1
  [C_LB_BMS_Status03_Timeout] -> Subsystem3/3(C_LB_BMS_Status03_Timeout)
  Demux/3 -> Terminator/1
  Demux/4 -> Terminator1/1
  Demux/5 -> Terminator2/1
  Demux/6 -> Terminator3/1
  Demux/7 -> Terminator4/1
  Demux/8 -> Terminator5/1
